simulink model "ofdm"  (R2015a)
settings: Solver=ode45  StartTime=0.0  StopTime=10  FixedStep=1e-6  RelTol=1e-3
libraries: commchan3 x4, commutil2 x4, commdigbbndpm3 x4, commsink2 x2, commofdm x2, commrandsrc2 x1
settings Model: Creator=jessica.c13  LastModifiedBy=jessica.c13
settings OptimizationCC: BlockReduction=off  ConditionallyExecuteInputs=off  InlineParams=on
settings DebuggingCC: AlgebraicLoopMsg=error
settings HardwareCC: ProdHWDeviceType=ASIC/FPGA->ASIC/FPGA  ProdEqTarget=off

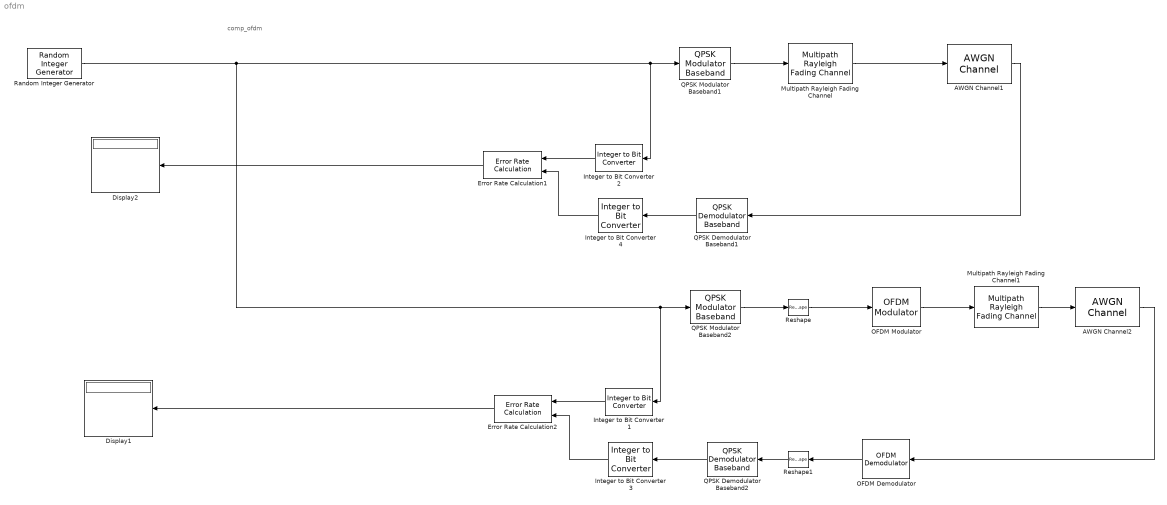
== system ofdm ==
  note: comp_ofdm
  AWGN Channel1 : commchan3/AWGN Channel  InputProcessing=Columns as channels (frame based)  seed=67  noiseMode="Signal to noise ratio  (SNR)"  EbNodB=10  EsNodB=10  SNRdB=10  bitsPerSym=1  Ps=1  Tsym=1  variance=1
  AWGN Channel2 : commchan3/AWGN Channel  InputProcessing=Columns as channels (frame based)  seed=67  noiseMode="Signal to noise ratio  (SNR)"  EbNodB=10  EsNodB=10  SNRdB=10  bitsPerSym=1  Ps=1  Tsym=1  variance=1
  Display1 : Display
  Display2 : Display
  Error Rate Calculation1 : commsink2/Error Rate Calculation  N=0  st_delay=0  cp_mode=Entire frame  subframe=[]  PMode=Port  WsName=e2  RsMode2=off  stop=off  numErr=100  maxBits=1e6
  Error Rate Calculation2 : commsink2/Error Rate Calculation  N=0  st_delay=0  cp_mode=Entire frame  subframe=[]  PMode=Port  WsName=e2  RsMode2=off  stop=off  numErr=100  maxBits=1e6
  Integer to Bit Converter {1..4} (4 alike) : commutil2/Integer to Bit Converter  nbits=2  signedInputValues=Unsigned  bitOrder=MSB first  outDtype=boolean
  Multipath Rayleigh Fading Channel : commchan3/Multipath Rayleigh Fading Channel  maxDopplerShift=600  spectrumType=Jakes  sigmaGaussian=1/sqrt(2)  coeffRounded=[1 -1.72 0.785]  freqMinMaxRJakes=[0 1]  freqMinMaxAJakes=[0 1]  sigmaGaussian1=1/sqrt(2)  sigmaGaussian2=1/sqrt(2)  centerFreqGaussian1=0.0  centerFreqGaussian2=0.0  gainGaussian1=0.5  gainGaussian2=0.5  coeffBell=9  dopplerSpectrum=doppler.jakes  pathDelays=[0 2e-6]  avgPathGaindB=[0 -3]  normalizePathGains=on  seed=73  enableProbe=0  openVisAtStart=off  outPathGains=off  outDelay=off
  Multipath Rayleigh Fading Channel1 : commchan3/Multipath Rayleigh Fading Channel  maxDopplerShift=600  spectrumType=Jakes  sigmaGaussian=1/sqrt(2)  coeffRounded=[1 -1.72 0.785]  freqMinMaxRJakes=[0 1]  freqMinMaxAJakes=[0 1]  sigmaGaussian1=1/sqrt(2)  sigmaGaussian2=1/sqrt(2)  centerFreqGaussian1=0.0  centerFreqGaussian2=0.0  gainGaussian1=0.5  gainGaussian2=0.5  coeffBell=9  dopplerSpectrum=doppler.jakes  pathDelays=[0 2e-6]  avgPathGaindB=[0 -3]  normalizePathGains=on  seed=73  enableProbe=0  openVisAtStart=off  outPathGains=off  outDelay=off
  OFDM Demodulator : commofdm/OFDM Demodulator  FFTLength=2048  NumGuardBandCarriers=[0; 0]  RemoveDCCarrier=off  PilotOutputPort=off  PilotCarrierIndices=[12; 26; 40; 54]  CyclicPrefixLength=16  NumSymbols=10  NumReceiveAntennas=1  SimulateUsing=Interpreted execution
  OFDM Modulator : commofdm/OFDM Modulator  FFTLength=2048  NumGuardBandCarriers=[0; 0]  InsertDCNull=off  PilotInputPort=off  PilotCarrierIndices=[12; 26; 40; 54]  CyclicPrefixLength=16  Windowing=off  WindowLength=1  NumSymbols=10  NumTransmitAntennas=1  SimulateUsing=Interpreted execution
  QPSK Demodulator Baseband1 : commdigbbndpm3/QPSK Demodulator Baseband  Ph=pi/4  Dec=Gray  OutType=Integer  DecType=Hard decision  VarSource=Dialog  Variance=1  outDtype1=Inherit via internal rule  outDtype2=Inherit via internal rule  derotateFactorWordLen=16
  QPSK Demodulator Baseband2 : commdigbbndpm3/QPSK Demodulator Baseband  Ph=pi/4  Dec=Gray  OutType=Integer  DecType=Hard decision  VarSource=Dialog  Variance=1  outDtype1=Inherit via internal rule  outDtype2=Inherit via internal rule  derotateFactorWordLen=16
  QPSK Modulator Baseband1 : commdigbbndpm3/QPSK Modulator Baseband  InType=Integer  Enc=Gray  Ph=pi/4  outDtype=double  outWordLen=16  outUDDataType=sfix(16)  outFracLenMode=Best precision  outFracLen=15
  QPSK Modulator Baseband2 : commdigbbndpm3/QPSK Modulator Baseband  InType=Integer  Enc=Gray  Ph=pi/4  outDtype=double  outWordLen=16  outUDDataType=sfix(16)  outFracLenMode=Best precision  outFracLen=15
  Random Integer Generator : commrandsrc2/Random Integer Generator  mul=3  seed=37  Ts=1/100000  frameBased=on  sampPerFrame=20480  orient=off  outDataType=double
  Reshape : Reshape  OutputDimensionality=Customize  OutputDimensions=[2048,10]
  Reshape1 : Reshape  OutputDimensionality=Customize  OutputDimensions=[20480,1]
  wires:
  Error Rate Calculation1/1 -> Display2/1
  Error Rate Calculation2/1 -> Display1/1
  Integer to Bit Converter 4/1 -> Error Rate Calculation1/2
  QPSK Demodulator Baseband1/1 -> Integer to Bit Converter 4/1
  QPSK Demodulator Baseband2/1 -> Integer to Bit Converter 3/1
  AWGN Channel2/1 -> OFDM Demodulator/1
  AWGN Channel1/1 -> QPSK Demodulator Baseband1/1
  Random Integer Generator/1 -> Integer to Bit Converter 1/1, QPSK Modulator Baseband2/1, Integer to Bit Converter 2/1, QPSK Modulator Baseband1/1
  Integer to Bit Converter 3/1 -> Error Rate Calculation2/2
  Integer to Bit Converter 1/1 -> Error Rate Calculation2/1
  Integer to Bit Converter 2/1 -> Error Rate Calculation1/1
  QPSK Modulator Baseband1/1 -> Multipath Rayleigh Fading Channel/1
  Multipath Rayleigh Fading Channel/1 -> AWGN Channel1/1
  Reshape1/1 -> QPSK Demodulator Baseband2/1
  Reshape/1 -> OFDM Modulator/1
  OFDM Demodulator/1 -> Reshape1/1
  QPSK Modulator Baseband2/1 -> Reshape/1
  Multipath Rayleigh Fading Channel1/1 -> AWGN Channel2/1
  OFDM Modulator/1 -> Multipath Rayleigh Fading Channel1/1
